simulink model "three_phase_inverter_igbt"  (R2024b)
settings: Solver=ode3  StartTime=0.0  StopTime=0.4  FixedStep=10e-6  RelTol=1e-3
model workspace (MAT data in the model file):
  pulse_generator_period = 0.02
libraries: spsIGBTLib x6, spsCurrentMeasurementLib x3, spsSeriesRLCLoadLib x3, spsVoltageMeasurementLib x3, spsDCVoltageSourceLib x1, sps_lib x1
settings Model: Creator=Abhijith_Kumble  LastModifiedBy=Abhijith_Kumble

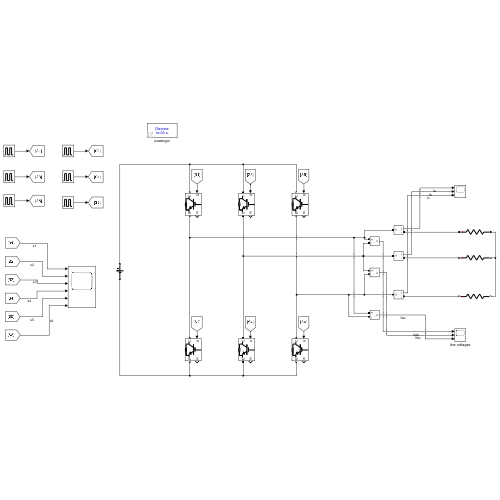
[thumbnail: Simulink's stored preview of the top-level diagram]
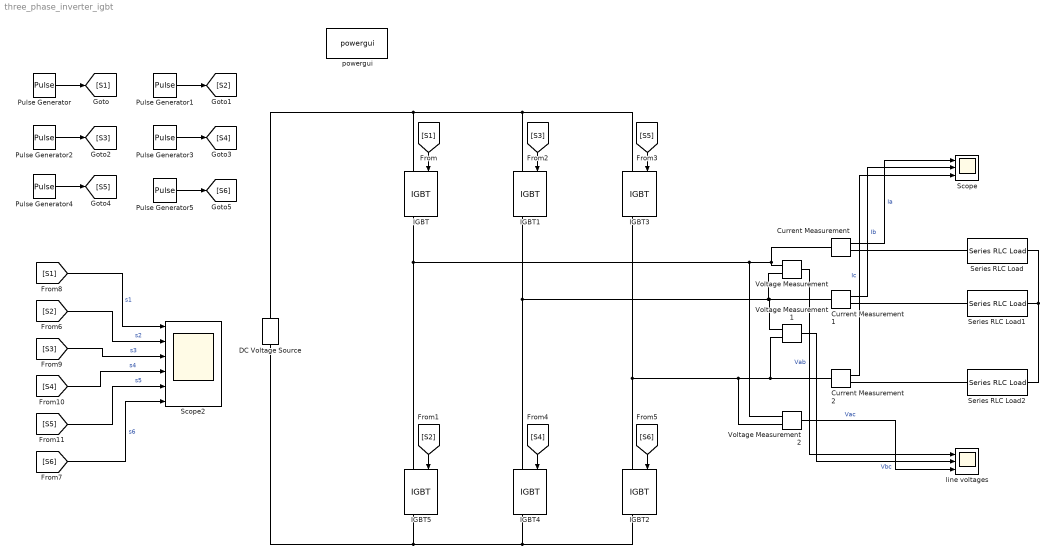
== system three_phase_inverter_igbt ==
  Current Measurement : spsCurrentMeasurementLib/Current Measurement  PhasorSimulation=off  OutputType=Complex  PSBequivalent=0
  Current Measurement1 : spsCurrentMeasurementLib/Current Measurement  PhasorSimulation=off  OutputType=Complex  PSBequivalent=0
  Current Measurement2 : spsCurrentMeasurementLib/Current Measurement  PhasorSimulation=off  OutputType=Complex  PSBequivalent=0
  DC Voltage Source : spsDCVoltageSourceLib/DC Voltage Source  Amplitude=415  Measurements=None
  IGBT{,1..5} (6 alike) : spsIGBTLib/IGBT  Ron=0.001  Lon=0  Vf=1  Tf=1e-6  Tt=2e-6  IC=0  Rs=1e5  Cs=inf  Measurements=on
  Pulse Generator : DiscretePulseGenerator  PulseType=Time based  Period=pulse_generator_period  PulseWidth=50
  Pulse Generator1 : DiscretePulseGenerator  PulseType=Time based  Period=pulse_generator_period  PulseWidth=50  PhaseDelay=13.3e-3
  Pulse Generator2 : DiscretePulseGenerator  PulseType=Time based  Period=pulse_generator_period  PulseWidth=50  PhaseDelay=6.67e-3
  Pulse Generator3 : DiscretePulseGenerator  PulseType=Time based  Period=pulse_generator_period  PulseWidth=50
  Pulse Generator4 : DiscretePulseGenerator  PulseType=Time based  Period=pulse_generator_period  PulseWidth=50  PhaseDelay=13.3e-3
  Pulse Generator5 : DiscretePulseGenerator  PulseType=Time based  Period=pulse_generator_period  PulseWidth=50  PhaseDelay=6.67e-3
  Scope : Scope  NumInputPorts=3
  Scope2 : Scope  NumInputPorts=6
  Series RLC Load : spsSeriesRLCLoadLib/Series RLC Load  LConnTagsString=a  RConnTagsString=__new0  NominalVoltage=1000  NominalFrequency=60  ActivePower=10e3  InductivePower=0  CapacitivePower=0  Setx0=off  InitialVoltage=0  SetiL0=off  InitialCurrent=0  Measurements=None  LoadType=constant Z
  Series RLC Load1 : spsSeriesRLCLoadLib/Series RLC Load  LConnTagsString=a  RConnTagsString=__new0  NominalVoltage=1000  NominalFrequency=60  ActivePower=10e3  InductivePower=0  CapacitivePower=0  Setx0=off  InitialVoltage=0  SetiL0=off  InitialCurrent=0  Measurements=None  LoadType=constant Z
  Series RLC Load2 : spsSeriesRLCLoadLib/Series RLC Load  LConnTagsString=a  RConnTagsString=__new0  NominalVoltage=1000  NominalFrequency=60  ActivePower=10e3  InductivePower=0  CapacitivePower=0  Setx0=off  InitialVoltage=0  SetiL0=off  InitialCurrent=0  Measurements=None  LoadType=constant Z
  Voltage Measurement : spsVoltageMeasurementLib/Voltage Measurement  PhasorSimulation=off  OutputType=Complex  PSBequivalent=0
  Voltage Measurement1 : spsVoltageMeasurementLib/Voltage Measurement  PhasorSimulation=off  OutputType=Complex  PSBequivalent=0
  Voltage Measurement2 : spsVoltageMeasurementLib/Voltage Measurement  PhasorSimulation=off  OutputType=Complex  PSBequivalent=0
  line voltages : Scope  NumInputPorts=3
  powergui : sps_lib/powergui  Priority=1  SimulationMode=Discrete  SampleTime=10e-6  frequency=60  Iterations=50  frequencyindice=0  Pbase=100e6  ErrMax=1e-4  UnitsV=kV  UnitsW=MW  buscounter=0  FunctionMessages=off  echomessages=off  EnableUseOfTLC=off  CurrentSourceSwitches=off  DisableSnubberDevices=off  DisableRonSwitches=off  DisableVfSwitches=off  DisplayEquations=off  AutomaticDiscreteSolvers=off  SolverType=Tustin/Backward Euler (TBE)  Interpol=off  ExternalGateDelay=off  methode=off  Ts=100  x0status=blocks  SPID=on  SwTol=0  HookPort=off  NonlinearTolerance=1e-4  nMaxIteration=100  ContinueOnMaxIteration=off  RestoreLinks=warning  ResistiveCurrentMeasurement=off  Frange=[0:2:500]  Ylog=off  Xlog=on  ShowGrid=off  save=off  variable=ZData  structure=0  ZoomFFT=off  StartTime=0.0  cycles=1  DisplayStyle=1  fundamental=60  FreqAxis=off  MaxFrequency=1000  frequencyindicesteady=1  RmsSteady=1  display=off
  wires:
  Current Measurement/1 -> Scope/1  "Ia"
  Current Measurement1/1 -> Scope/2  "Ib"
  Current Measurement2/1 -> Scope/3  "Ic"
  Voltage Measurement/1 -> line voltages/1  "Vab"
  Voltage Measurement1/1 -> line voltages/2  "Vbc"
  Voltage Measurement2/1 -> line voltages/3  "Vac"
  Pulse Generator/1 -> [S1]
  [S1] -> IGBT/1
  [S2] -> IGBT5/1
  [S3] -> IGBT1/1
  [S5] -> IGBT3/1
  [S4] -> IGBT4/1
  [S6] -> IGBT2/1
  Pulse Generator1/1 -> [S2]
  Pulse Generator2/1 -> [S3]
  Pulse Generator4/1 -> [S5]
  Pulse Generator3/1 -> [S4]
  Pulse Generator5/1 -> [S6]
  [S1] -> Scope2/1  "s1"
  [S2] -> Scope2/2  "s2"
  [S3] -> Scope2/3  "s3"
  [S4] -> Scope2/4  "s4"
  [S5] -> Scope2/5  "s5"
  [S6] -> Scope2/6  "s6"
  connections:
  IGBT/RConn1 -- IGBT5/LConn1 -- Voltage Measurement2/LConn1 -- Current Measurement/LConn1 -- Voltage Measurement/LConn1
  IGBT1/RConn1 -- IGBT4/LConn1 -- Voltage Measurement1/LConn1 -- Current Measurement1/LConn1 -- Voltage Measurement/LConn2
  IGBT3/RConn1 -- IGBT2/LConn1 -- Voltage Measurement2/LConn2 -- Voltage Measurement1/LConn2 -- Current Measurement2/LConn1
  DC Voltage Source/RConn1 -- IGBT3/LConn1 -- IGBT1/LConn1 -- IGBT/LConn1
  DC Voltage Source/LConn1 -- IGBT2/RConn1 -- IGBT4/RConn1 -- IGBT5/RConn1
  Series RLC Load/RConn1 -- Series RLC Load2/RConn1 -- Series RLC Load1/RConn1
  Current Measurement/RConn1 -- Series RLC Load/LConn1
  Series RLC Load1/LConn1 -- Current Measurement1/RConn1
  Current Measurement2/RConn1 -- Series RLC Load2/LConn1
